simulink model "robust_tracking_digital_filtered"  (R2021b)
settings: Solver=ode15s  StartTime=0.0  StopTime=10  RelTol=1e-3
undefined symbols (not defined in the file): ball, ballnbeam, const, driver, mech, sensor, stepper
libraries: simulink x1
settings Model: Creator=Utente  LastModifiedBy=Utente
settings SolverCC: AlgebraicLoopSolver=TrustRegion
settings DebuggingCC: SFMachineParentedDataDiag=warning

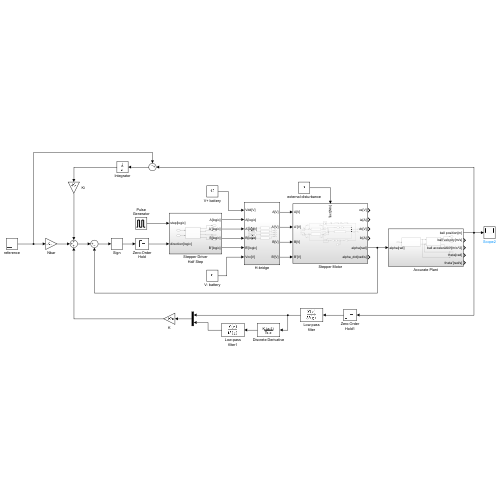
[thumbnail: Simulink's stored preview of the top-level diagram]
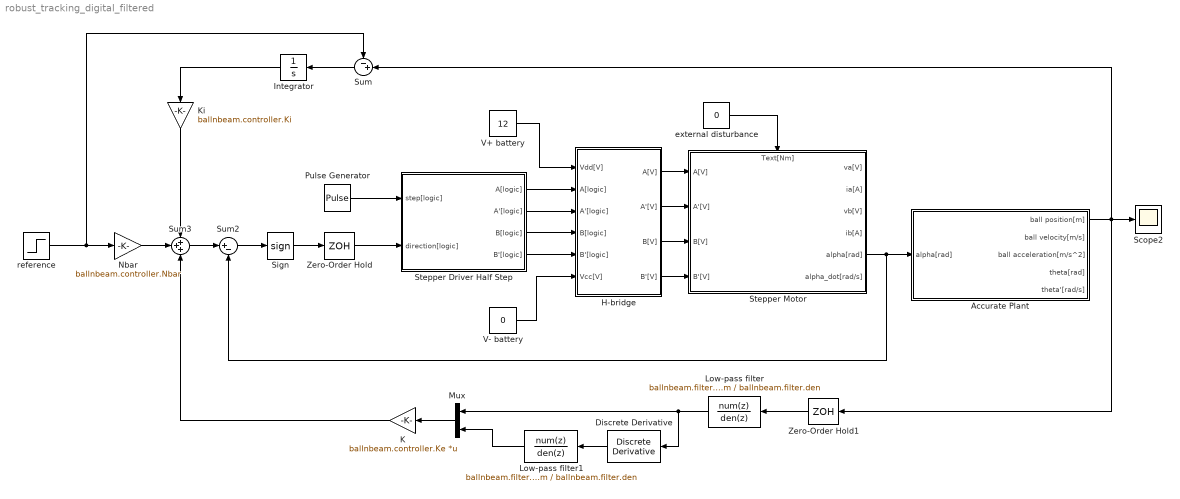
== system robust_tracking_digital_filtered ==
  Accurate Plant : Subsystem
  Discrete Derivative : simulink/Discrete/Discrete Derivative  gainval=1.0  ICPrevScaledInput=0.0  OutMin=[]  OutMax=[]  OutDataType=fixdt(1, 16)  OutScaling=2^-10  DoSatur=off
  H-bridge : Subsystem
  Integrator : Integrator
  K : Gain  Gain=ballnbeam.controller.Ke  Multiplication=Matrix(K*u)
  Ki : Gain  Gain=ballnbeam.controller.Ki
  Low-pass filter : DiscreteTransferFcn  Numerator=ballnbeam.filter.num  Denominator=ballnbeam.filter.den  SampleTime=sensor.distance.Ts
  Low-pass filter1 : DiscreteTransferFcn  Numerator=ballnbeam.filter.num  Denominator=ballnbeam.filter.den  SampleTime=sensor.distance.Ts
  Mux : Mux  Inputs=2
  Nbar : Gain  Gain=ballnbeam.controller.Nbar
  Pulse Generator : DiscretePulseGenerator  PulseType=Time based  Period=stepper.Tstep2  PulseWidth=50
  Scope2 : Scope
  Sign : Signum
  Stepper Driver Half Step : Subsystem
  Stepper Motor : Subsystem
      settings: PortSchema="{\"entries\":[{\"content\":{\"sides\":[{\"content\":{\"connectorIds\":[\"In1\",\"In2\",\"In3\",\"In4\"]},\"type\":\"ConnectorPlacement.EquallySpacedRectSide\",\"uuid\":\"73295f7e-2188-4526-b3fe-31d6eab8afcb\"},{\"content\":{\"connectorIds\":[\"Out1\",\"Out2\",\"Out3\",\"Out4\",\"Out5\",\"Out6\"],\"side\":\"RIGHT\"},\"type\":\"ConnectorPlacement.EquallySpacedRectSide\",\"uuid\":\"77dcaa74-ce65-4a13-97c5-e825e2410182\"},{\"content\":{\"connectorIds\":[\"In5\"],\"side\":\"TOP\"},\"type\":\"ConnectorPlacement.EquallySpacedRectSide\",\"uuid\":\"bac6b674-d00a-4490-8f08-a2567c8e6873\"},{\"content\":{\"connectorIds\":[],\"side\":\"HIDDEN\"},\"type\":\"ConnectorPlacement.EquallySpacedRectSide\",\"uuid\":\"66c41dc0-366a-490c-a787-062f795e6cc7\"}]},\"type\":\"ConnectorPlacement.EquallySpacedConnector\",\"uuid\":\"3c22aa21-f88d-4b07-855c-a69922a8689b\"}],\"packageUris\":[\"http://schema.mathworks.com/mf0/Connector/R2020b\"],\"version\":\"1.0\"}"
  Sum : Sum  Inputs=-+|
  Sum2 : Sum  Inputs=|+-
  Sum3 : Sum  Inputs=+++
  V+ battery : Constant  Value=12
  V- battery : Constant  Value=0
  Zero-Order Hold : ZeroOrderHold  SampleTime=sensor.distance.Ts
  Zero-Order Hold1 : ZeroOrderHold  SampleTime=sensor.distance.Ts
  external disturbance : Constant  Value=0
  reference : Step  Time=0  After=0.25  SampleTime=0
  wires:
  reference/1 -> Sum/1, Nbar/1
  Nbar/1 -> Sum3/2
  K/1 -> Sum3/3
  Ki/1 -> Sum3/1
  Integrator/1 -> Ki/1
  Sum/1 -> Integrator/1
  Stepper Motor/5(alpha[rad]) -> Accurate Plant/1(alpha[rad]), Sum2/2
  H-bridge/2(A'[V]) -> Stepper Motor/2(A'[V])
  external disturbance/1 -> Stepper Motor/5(Text[Nm])
  H-bridge/4(B'[V]) -> Stepper Motor/4(B'[V])
  Stepper Driver Half Step/4(B'[logic]) -> H-bridge/5(B'[logic])
  Stepper Driver Half Step/2(A'[logic]) -> H-bridge/3(A'[logic])
  Sum2/1 -> Sign/1
  V+ battery/1 -> H-bridge/1(Vdd[V])
  Stepper Driver Half Step/3(B[logic]) -> H-bridge/4(B[logic])
  Stepper Driver Half Step/1(A[logic]) -> H-bridge/2(A[logic])
  Sum3/1 -> Sum2/1
  H-bridge/3(B[V]) -> Stepper Motor/3(B[V])
  Pulse Generator/1 -> Stepper Driver Half Step/1(step[logic])
  H-bridge/1(A[V]) -> Stepper Motor/1(A[V])
  Sign/1 -> Zero-Order Hold/1
  V- battery/1 -> H-bridge/6(Vcc[V])
  Zero-Order Hold/1 -> Stepper Driver Half Step/2(direction[logic])
  Zero-Order Hold1/1 -> Low-pass filter/1
  Low-pass filter1/1 -> Mux/2
  Mux/1 -> K/1
  Accurate Plant/1(ball position[m]) -> Scope2/1, Sum/2, Zero-Order Hold1/1
  Low-pass filter/1 -> Mux/1, Discrete Derivative/1
  Discrete Derivative/1 -> Low-pass filter1/1

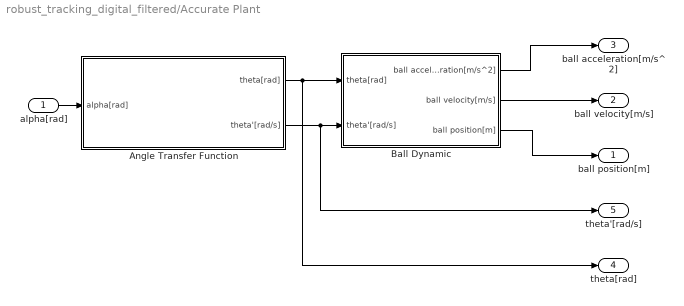
== system robust_tracking_digital_filtered/Accurate Plant ==
  alpha[rad] : Inport
  Angle Transfer Function : Subsystem
  Ball Dynamic : Subsystem
  ball position[m] : Outport
  ball velocity[m/s] : Outport  Port=2
  ball acceleration[m/s^2] : Outport  Port=3
  theta[rad] : Outport  Port=4
  theta'[rad/s] : Outport  Port=5
  wires:
  alpha[rad]/1 -> Angle Transfer Function/1(alpha[rad])
  Angle Transfer Function/1(theta[rad]) -> theta[rad]/1, Ball Dynamic/1(theta[rad])
  Angle Transfer Function/2(theta'[rad/s]) -> Ball Dynamic/2(theta'[rad/s]), theta'[rad/s]/1
  Ball Dynamic/2(ball velocity[m/s]) -> ball velocity[m/s]/1
  Ball Dynamic/1(ball acceleration[m/s^2]) -> ball acceleration[m/s^2]/1
  Ball Dynamic/3(ball position[m]) -> ball position[m]/1

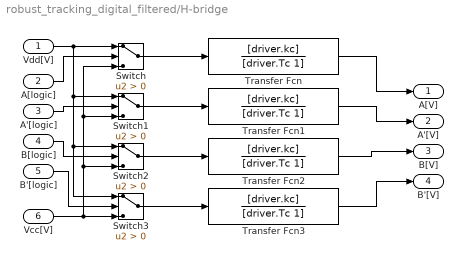
== system robust_tracking_digital_filtered/H-bridge ==
  Vdd[V] : Inport
  A[logic] : Inport  Port=2
  A'[logic] : Inport  Port=3
  B[logic] : Inport  Port=4
  B'[logic] : Inport  Port=5
  Vcc[V] : Inport  Port=6
  Switch{,1..3} (4 alike) : Switch  Criteria=u2 > Threshold
  Transfer Fcn{,1..3} (4 alike) : TransferFcn  Numerator=[driver.kc]  Denominator=[driver.Tc 1]
  A[V] : Outport
  A'[V] : Outport  Port=2
  B[V] : Outport  Port=3
  B'[V] : Outport  Port=4
  wires:
  Vcc[V]/1 -> Switch/3, Switch1/3, Switch2/3, Switch3/3
  A'[logic]/1 -> Switch1/2
  A[logic]/1 -> Switch/2
  B'[logic]/1 -> Switch3/2
  Vdd[V]/1 -> Switch3/1, Switch2/1, Switch1/1, Switch/1
  B[logic]/1 -> Switch2/2
  Switch/1 -> Transfer Fcn/1
  Switch3/1 -> Transfer Fcn3/1
  Switch2/1 -> Transfer Fcn2/1
  Switch1/1 -> Transfer Fcn1/1
  Transfer Fcn2/1 -> B[V]/1
  Transfer Fcn1/1 -> A'[V]/1
  Transfer Fcn/1 -> A[V]/1
  Transfer Fcn3/1 -> B'[V]/1

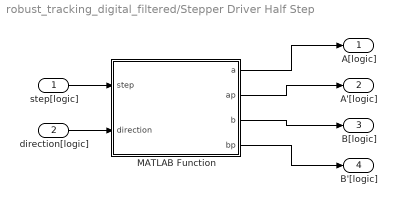
== system robust_tracking_digital_filtered/Stepper Driver Half Step ==
  step[logic] : Inport
  direction[logic] : Inport  Port=2
  MATLAB Function : MATLAB Function  TreatAsAtomicUnit=on
  A[logic] : Outport
  A'[logic] : Outport  Port=2
  B[logic] : Outport  Port=3
  B'[logic] : Outport  Port=4
  wires:
  step[logic]/1 -> MATLAB Function/1(step)
  direction[logic]/1 -> MATLAB Function/2(direction)
  MATLAB Function/2(ap) -> A'[logic]/1
  MATLAB Function/1(a) -> A[logic]/1
  MATLAB Function/3(b) -> B[logic]/1
  MATLAB Function/4(bp) -> B'[logic]/1

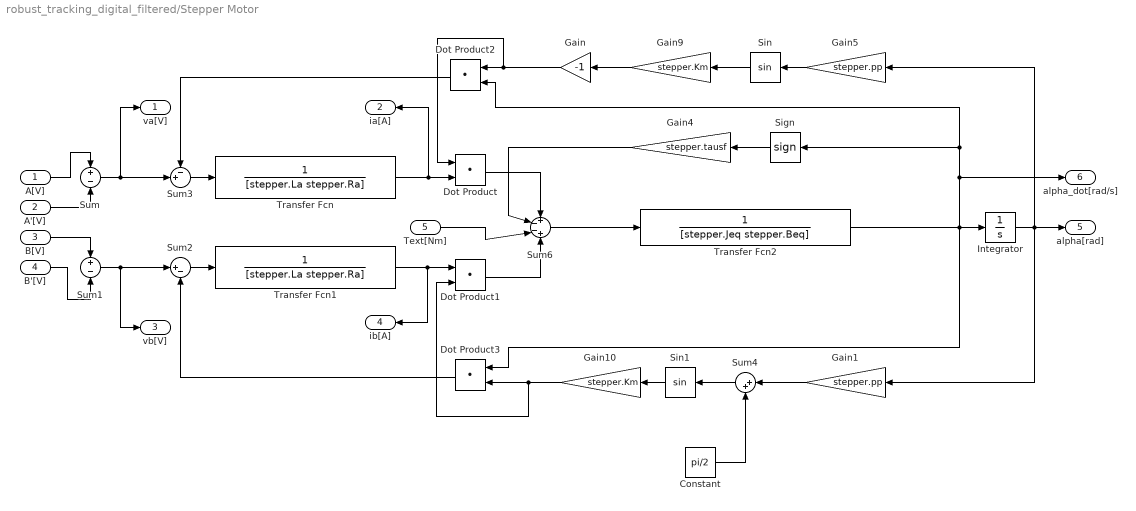
== system robust_tracking_digital_filtered/Stepper Motor ==
  A[V] : Inport
  A'[V] : Inport  Port=2
  B[V] : Inport  Port=3
  B'[V] : Inport  Port=4
  Text[Nm] : Inport  Port=5
  Constant : Constant  Value=pi/2
  Dot Product{,1..3} (4 alike) : DotProduct  InputSameDT=on  OutDataTypeStr=Inherit: Inherit via internal rule
  Gain : Gain  Gain=-1
  Gain1 : Gain  Gain=stepper.pp
  Gain10 : Gain  Gain=stepper.Km
  Gain4 : Gain  Gain=stepper.tausf
  Gain5 : Gain  Gain=stepper.pp
  Gain9 : Gain  Gain=stepper.Km
  Integrator : Integrator
  Sign : Signum
  Sin : Trigonometry
  Sin1 : Trigonometry
  Sum : Sum  Inputs=+|-
  Sum1 : Sum  Inputs=+|-
  Sum2 : Sum  Inputs=|+-
  Sum3 : Sum  Inputs=-+|
  Sum4 : Sum  Inputs=|++
  Sum6 : Sum  Inputs=+--+
  Transfer Fcn : TransferFcn  Denominator=[stepper.La stepper.Ra]
  Transfer Fcn1 : TransferFcn  Denominator=[stepper.La stepper.Ra]
  Transfer Fcn2 : TransferFcn  Denominator=[stepper.Jeq stepper.Beq]
  va[V] : Outport
  ia[A] : Outport  Port=2
  vb[V] : Outport  Port=3
  ib[A] : Outport  Port=4
  alpha[rad] : Outport  Port=5
  alpha_dot[rad/s] : Outport  Port=6
  wires:
  A'[V]/1 -> Sum/2
  A[V]/1 -> Sum/1
  Sum/1 -> Sum3/2, va[V]/1
  B[V]/1 -> Sum1/1
  B'[V]/1 -> Sum1/2
  Sum1/1 -> Sum2/1, vb[V]/1
  Sum3/1 -> Transfer Fcn/1
  Sum2/1 -> Transfer Fcn1/1
  Dot Product/1 -> Sum6/1
  Sum6/1 -> Transfer Fcn2/1
  Gain4/1 -> Sum6/2
  Transfer Fcn/1 -> Dot Product/2, ia[A]/1
  Transfer Fcn1/1 -> ib[A]/1, Dot Product1/1
  Gain5/1 -> Sin/1
  Integrator/1 -> Gain1/1, Gain5/1, alpha[rad]/1
  Transfer Fcn2/1 -> Dot Product3/1, Dot Product2/2, Sign/1, alpha_dot[rad/s]/1, Integrator/1
  Sin/1 -> Gain9/1
  Sin1/1 -> Gain10/1
  Dot Product3/1 -> Sum2/2
  Dot Product2/1 -> Sum3/1
  Gain10/1 -> Dot Product1/2, Dot Product3/2
  Sign/1 -> Gain4/1
  Gain9/1 -> Gain/1
  Dot Product1/1 -> Sum6/4
  Sum4/1 -> Sin1/1
  Gain1/1 -> Sum4/1
  Constant/1 -> Sum4/2
  Gain/1 -> Dot Product/1, Dot Product2/1
  Text[Nm]/1 -> Sum6/3

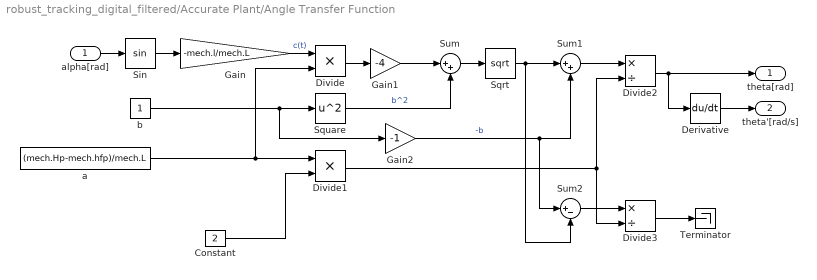
== system robust_tracking_digital_filtered/Accurate Plant/Angle Transfer Function ==
  alpha[rad] : Inport
  Constant : Constant  Value=2
  Derivative : Derivative
  Divide : Product  Inputs=**
  Divide1 : Product  Inputs=**
  Divide2 : Product  Inputs=*/
  Divide3 : Product  Inputs=*/
  Gain : Gain  Gain=-mech.l/mech.L
  Gain1 : Gain  Gain=-4
  Gain2 : Gain  Gain=-1
  Sin : Trigonometry
  Sqrt : Sqrt  SaturateOnIntegerOverflow=on
  Square : Math  Operator=square  SaturateOnIntegerOverflow=on
  Sum : Sum  Inputs=|++
  Sum1 : Sum  Inputs=|++
  Sum2 : Sum  Inputs=|+-
  Terminator : Terminator
  a : Constant  Value=(mech.Hp-mech.hfp)/mech.L
  b : Constant
  theta[rad] : Outport
  theta'[rad/s] : Outport  Port=2
  wires:
  alpha[rad]/1 -> Sin/1
  Sin/1 -> Gain/1
  Divide/1 -> Gain1/1
  Gain/1 -> Divide/1  "c(t)"
  a/1 -> Divide/2, Divide1/1
  b/1 -> Gain2/1, Square/1
  Sum/1 -> Sqrt/1
  Gain1/1 -> Sum/1
  Square/1 -> Sum/2  "b^2"
  Constant/1 -> Divide1/2
  Gain2/1 -> Sum2/1, Sum1/2  "-b"
  Sqrt/1 -> Sum1/1, Sum2/2
  Sum1/1 -> Divide2/1
  Divide1/1 -> Divide3/2, Divide2/2
  Sum2/1 -> Divide3/1
  Divide3/1 -> Terminator/1
  Divide2/1 -> Derivative/1, theta[rad]/1
  Derivative/1 -> theta'[rad/s]/1

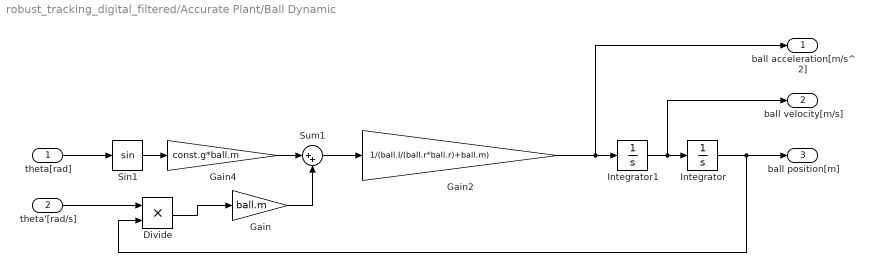
== system robust_tracking_digital_filtered/Accurate Plant/Ball Dynamic ==
  theta[rad] : Inport
  theta'[rad/s] : Inport  Port=2
  Divide : Product  Inputs=**
  Gain : Gain  Gain=ball.m
  Gain2 : Gain  Gain=1/(ball.I/(ball.r*ball.r)+ball.m)
  Gain4 : Gain  Gain=const.g*ball.m
  Integrator : Integrator
  Integrator1 : Integrator
  Sin1 : Trigonometry
  Sum1 : Sum  Inputs=|++
  ball acceleration[m/s^2] : Outport
  ball velocity[m/s] : Outport  Port=2
  ball position[m] : Outport  Port=3
  wires:
  Integrator1/1 -> ball velocity[m/s]/1, Integrator/1
  Gain/1 -> Sum1/2
  Integrator/1 -> Divide/2, ball position[m]/1
  Sin1/1 -> Gain4/1
  Sum1/1 -> Gain2/1
  Gain2/1 -> ball acceleration[m/s^2]/1, Integrator1/1
  Gain4/1 -> Sum1/1
  theta[rad]/1 -> Sin1/1
  Divide/1 -> Gain/1
  theta'[rad/s]/1 -> Divide/1

== matlab function robust_tracking_digital_filtered/Stepper Driver Half Step/MATLAB Function ==
  data: step input; a output; direction input; ap output; b output; bp output
function [a,ap,b,bp]= fcn(step, direction)
    lookup = [[1,0,1,0];[0,0,1,0];[0,1,1,0];[0,1,0,0];[0,1,0,1];[0,0,0,1];[1,0,0,1];[1,0,0,0]];
    persistent i;  % index on the lookup table
    persistent x;  % last output command (hold)
    persistent st; % previous step command
    % initial conditions
    if isempty(i)
        i = 0;
    end
    if isempty(x)
        x = [0,0,0,0];
    end
    if isempty(st)
        st = 0;
    end
    % function
    if step == 1 && st == 0
        if direction == 1
            if i + 1 >= 9
                i = 0;
            end
            i = i + 1;
            x = lookup(i,1:4);
        end
        if direction == -1
            if i - 1 <= 0
                i = 9;
            end
            i = i - 1;
            x = lookup(i,1:4);
        end
    else
        %x = [0,0,0,0];
    end
    % set persistent state and output
    st = step;
    a=x(1);
    ap=x(2);
    b=x(3);
    bp=x(4);
end
